simulink model "TEP_Final_NoScript"  (R2024a)
settings: Solver=FixedStepAuto  StartTime=0.0  StopTime=10  FixedStep=1/3600  RelTol=1e-3
model workspace (MAT data in the model file):
  AD : Simulink.Parameter (value not decoded)
  AG : Simulink.Parameter (value not decoded)
  AH : Simulink.Parameter (value not decoded)
  AV : Simulink.Parameter (value not decoded)
  AVP : Simulink.Parameter (value not decoded)
  BCHL : Simulink.Parameter (value not decoded)
  BCHV : Simulink.Parameter (value not decoded)
  BD : Simulink.Parameter (value not decoded)
  BG : Simulink.Parameter (value not decoded)
  BH : Simulink.Parameter (value not decoded)
  BVP : Simulink.Parameter (value not decoded)
  CD : Simulink.Parameter (value not decoded)
  CG : Simulink.Parameter (value not decoded)
  CH : Simulink.Parameter (value not decoded)
  CVP : Simulink.Parameter (value not decoded)
  XMW : Simulink.Parameter (value not decoded)
  XNS : Simulink.Parameter (value not decoded)
  XNSE : Simulink.Parameter (value not decoded)
symbols that are objects in the model workspace (value not decoded): AD, AG, AH, AV, AVP, BD, BG, BH, BVP, CD, CG, CH, CVP, XMW, XNS, XNSE
undefined symbols (not defined in the file or in its folder): magnitude, msgbox, SETPT, XMEAS, XMV
libraries: mylib x360, dspindex x28
(part 5 of 14)

== system TEP_Final_NoScript/Mixing Zone/Holdup of Components in Mixing Zone/Subsystem ==
  Properties of Stream 1 : Inport
  Bus Creator : BusCreator  Inputs=8
  Bus Selector : BusSelector  OutputSignals=FCM(I;1)
  Multiport Selector : dspindex/Multiport Selector  rowsOrCols=Rows  idxCellArray={ 1,2,3,4,5,6,7,8}  idxErrMode=Clip Index
  FCM(I;1) : Outport  VectorParamsAs1DForOutWhenUnconnected=off
  wires:
  Multiport Selector/1 -> Bus Creator/1  "FCM(1;1)"
  Multiport Selector/2 -> Bus Creator/2  "FCM(2;1)"
  Multiport Selector/8 -> Bus Creator/8  "FCM(8;1)"
  Multiport Selector/6 -> Bus Creator/6  "FCM(6;1)"
  Multiport Selector/7 -> Bus Creator/7  "FCM(7;1)"
  Multiport Selector/4 -> Bus Creator/4  "FCM(4;1)"
  Multiport Selector/5 -> Bus Creator/5  "FCM(5;1)"
  Multiport Selector/3 -> Bus Creator/3  "FCM(3;1)"
  Bus Selector/1 -> Multiport Selector/1  "<FCM(I;1)>"
  Properties of Stream 1/1 -> Bus Selector/1
  Bus Creator/1 -> FCM(I;1)/1

== system TEP_Final_NoScript/Mixing Zone/Holdup of Components in Mixing Zone/Subsystem1 ==
  Properties of Stream 2 : Inport
  Bus Creator : BusCreator  Inputs=8
  Bus Selector1 : BusSelector  OutputSignals=FCM(I;2)
  Multiport Selector1 : dspindex/Multiport Selector  rowsOrCols=Rows  idxCellArray={ 1,2,3,4,5,6,7,8}  idxErrMode=Clip Index
  FCM(I;2) : Outport  VectorParamsAs1DForOutWhenUnconnected=off
  wires:
  Multiport Selector1/5 -> Bus Creator/5  "FCM(5;2)"
  Bus Selector1/1 -> Multiport Selector1/1  "<FCM(I;2)>"
  Multiport Selector1/6 -> Bus Creator/6  "FCM(6;2)"
  Multiport Selector1/1 -> Bus Creator/1  "FCM(1;2)"
  Multiport Selector1/2 -> Bus Creator/2  "FCM(2;2)"
  Multiport Selector1/7 -> Bus Creator/7  "FCM(7;2)"
  Multiport Selector1/4 -> Bus Creator/4  "FCM(4;2)"
  Multiport Selector1/8 -> Bus Creator/8  "FCM(8;2)"
  Multiport Selector1/3 -> Bus Creator/3  "FCM(3;2)"
  Properties of Stream 2/1 -> Bus Selector1/1
  Bus Creator/1 -> FCM(I;2)/1

== system TEP_Final_NoScript/Mixing Zone/Holdup of Components in Mixing Zone/Subsystem2 ==
  Bus Creator : BusCreator  Inputs=8
  Bus Selector5 : BusSelector  OutputSignals=signal1.FCM(I;6) = FCM(I;7)
  Multiport Selector4 : dspindex/Multiport Selector  rowsOrCols=Rows  idxCellArray={ 1,2,3,4,5,6,7,8}  idxErrMode=Clip Index
  FCM(I;6) : Outport  VectorParamsAs1DForOutWhenUnconnected=off
  wires:
  Multiport Selector4/6 -> Bus Creator/6  "FCM(6;7)"
  Multiport Selector4/7 -> Bus Creator/7  "FCM(7;7)"
  Multiport Selector4/5 -> Bus Creator/5  "FCM(5;7)"
  Multiport Selector4/4 -> Bus Creator/4  "FCM(4;7)"
  Multiport Selector4/8 -> Bus Creator/8  "FCM(8;7)"
  Multiport Selector4/3 -> Bus Creator/3  "FCM(3;7)"
  Multiport Selector4/2 -> Bus Creator/2  "FCM(2;7)"
  [PropertiesStream6] -> Bus Selector5/1
  Multiport Selector4/1 -> Bus Creator/1  "FCM(1;7)"
  Bus Selector5/1 -> Multiport Selector4/1  "<FCM(I;6) = FCM(I;7)>"
  Bus Creator/1 -> FCM(I;6)/1

== system TEP_Final_NoScript/Mixing Zone/Holdup of Components in Mixing Zone/Subsystem3 ==
  Properties of Stream 3 : Inport
  Bus Creator : BusCreator  Inputs=8
  Bus Selector2 : BusSelector  OutputSignals=FCM(I;3)
  Multiport Selector2 : dspindex/Multiport Selector  rowsOrCols=Rows  idxCellArray={ 1,2,3,4,5,6,7,8}  idxErrMode=Clip Index
  FCM(I;3) : Outport  VectorParamsAs1DForOutWhenUnconnected=off
  wires:
  Multiport Selector2/2 -> Bus Creator/2  "FCM(2;3)"
  Multiport Selector2/4 -> Bus Creator/4  "FCM(4;3)"
  Multiport Selector2/8 -> Bus Creator/8  "FCM(8;3)"
  Bus Selector2/1 -> Multiport Selector2/1  "<FCM(I;3)>"
  Multiport Selector2/7 -> Bus Creator/7  "FCM(7;3)"
  Multiport Selector2/6 -> Bus Creator/6  "FCM(6;3)"
  Multiport Selector2/1 -> Bus Creator/1  "FCM(1;3)"
  Multiport Selector2/3 -> Bus Creator/3  "FCM(3;3)"
  Multiport Selector2/5 -> Bus Creator/5  "FCM(5;3)"
  Properties of Stream 3/1 -> Bus Selector2/1
  Bus Creator/1 -> FCM(I;3)/1

== system TEP_Final_NoScript/Mixing Zone/Holdup of Components in Mixing Zone/Subsystem4 ==
  Properties of Stream 5 : Inport
  Bus Creator : BusCreator  Inputs=8
  Bus Selector3 : BusSelector  OutputSignals=FCM(I;5)
  Multiport Selector3 : dspindex/Multiport Selector  rowsOrCols=Rows  idxCellArray={ 1,2,3,4,5,6,7,8}  idxErrMode=Clip Index
  FCM(I;5) : Outport  VectorParamsAs1DForOutWhenUnconnected=off
  wires:
  Multiport Selector3/6 -> Bus Creator/6  "FCM(6;5)"
  Multiport Selector3/8 -> Bus Creator/8  "FCM(8;5)"
  Multiport Selector3/5 -> Bus Creator/5  "FCM(5;5)"
  Multiport Selector3/2 -> Bus Creator/2  "FCM(2;5)"
  Bus Selector3/1 -> Multiport Selector3/1  "<FCM(I;5)>"
  Multiport Selector3/7 -> Bus Creator/7  "FCM(7;5)"
  Multiport Selector3/4 -> Bus Creator/4  "FCM(4;5)"
  Multiport Selector3/1 -> Bus Creator/1  "FCM(1;5)"
  Multiport Selector3/3 -> Bus Creator/3  "FCM(3;5)"
  Properties of Stream 5/1 -> Bus Selector3/1
  Bus Creator/1 -> FCM(I;5)/1

== system TEP_Final_NoScript/Mixing Zone/Holdup of Components in Mixing Zone/Subsystem5 ==
  Properties of Stream 9 : Inport
  Bus Creator : BusCreator  Inputs=8
  Bus Selector4 : BusSelector  OutputSignals=FCM(I;9)
  Multiport Selector5 : dspindex/Multiport Selector  rowsOrCols=Rows  idxCellArray={ 1,2,3,4,5,6,7,8}  idxErrMode=Clip Index
  FCM(I;9) : Outport  VectorParamsAs1DForOutWhenUnconnected=off
  wires:
  Multiport Selector5/7 -> Bus Creator/7  "FCM(7;9)"
  Multiport Selector5/6 -> Bus Creator/6  "FCM(6;9)"
  Multiport Selector5/8 -> Bus Creator/8  "FCM(8;9)"
  Bus Selector4/1 -> Multiport Selector5/1  "<FCM(I;9)>"
  Multiport Selector5/1 -> Bus Creator/1  "FCM(1;9)"
  Multiport Selector5/2 -> Bus Creator/2  "FCM(2;9)"
  Multiport Selector5/5 -> Bus Creator/5  "FCM(5;9)"
  Multiport Selector5/4 -> Bus Creator/4  "FCM(4;9)"
  Multiport Selector5/3 -> Bus Creator/3  "FCM(3;9)"
  Properties of Stream 9/1 -> Bus Selector4/1
  Bus Creator/1 -> FCM(I;9)/1

== system TEP_Final_NoScript/Mixing Zone/Holdup of Components in Mixing Zone/Vapour Holdup Fraction in the Mxing Zone ==
  UTVV : Inport
  UCVV : Inport  Port=2
  Bus Selector : BusSelector  OutputSignals=UCVV(1),UCVV(2),UCVV(3),UCVV(4),UCVV(5),UCVV(6),UCVV(7),UCVV(8)
  Mux : Mux  Inputs=8
  XVV(1) : Product  Inputs=*/
  XVV(2) : Product  Inputs=*/
  XVV(3) : Product  Inputs=*/
  XVV(4) : Product  Inputs=*/
  XVV(5) : Product  Inputs=*/
  XVV(6) : Product  Inputs=*/
  XVV(7) : Product  Inputs=*/
  XVV(8) : Product  Inputs=*/
  XVV : Outport  VectorParamsAs1DForOutWhenUnconnected=off
  wires:
  XVV(4)/1 -> Mux/4  "XVV(4)"
  UTVV/1 -> XVV(8)/2, XVV(7)/2, XVV(6)/2, XVV(5)/2, XVV(4)/2, XVV(3)/2, XVV(2)/2, XVV(1)/2
  XVV(8)/1 -> Mux/8  "XVV(8)"
  Bus Selector/3 -> XVV(3)/1  "<UCVV(3)>"
  XVV(5)/1 -> Mux/5  "XVV(5)"
  XVV(2)/1 -> Mux/2  "XVV(2)"
  XVV(7)/1 -> Mux/7  "XVV(7)"
  Bus Selector/8 -> XVV(8)/1  "<UCVV(8)>"
  XVV(6)/1 -> Mux/6  "XVV(6)"
  XVV(3)/1 -> Mux/3  "XVV(3)"
  Mux/1 -> XVV/1
  XVV(1)/1 -> Mux/1  "XVV(1)"
  Bus Selector/7 -> XVV(7)/1  "<UCVV(7)>"
  Bus Selector/5 -> XVV(5)/1  "<UCVV(5)>"
  Bus Selector/4 -> XVV(4)/1  "<UCVV(4)>"
  Bus Selector/2 -> XVV(2)/1  "<UCVV(2)>"
  Bus Selector/6 -> XVV(6)/1  "<UCVV(6)>"
  UCVV/1 -> Bus Selector/1
  Bus Selector/1 -> XVV(1)/1  "<UCVV(1)>"

== system TEP_Final_NoScript/Mixing Zone/Holdup of Components in Mixing Zone/YP(28) ==
  FCM(1,1) : Inport
  FCM(1,2) : Inport  Port=2
  FCM(1,3) : Inport  Port=3
  FCM(1,5) : Inport  Port=4
  FCM(1,9) : Inport  Port=5
  FCM(1,6) : Inport  Port=6
  " " : Sum  Inputs=+++++-
  Bus Selector : BusSelector  OutputSignals=FCM(1;1)
  Bus Selector1 : BusSelector  OutputSignals=FCM(1;2)
  Bus Selector2 : BusSelector  OutputSignals=FCM(1;3)
  Bus Selector3 : BusSelector  OutputSignals=FCM(1;5)
  Bus Selector4 : BusSelector  OutputSignals=FCM(1;9)
  Bus Selector5 : BusSelector  OutputSignals=FCM(1;7)
  Integration : mylib/Integration  SystemSampleTime=-1  VariantActivationTime=update diagram  AllowFlexibleInterface=on  Latency=0  AutoFrameSizeCalculation=off
      settings: SourceProductName=TEP Library
  "YY(28) " : Constant  Value=107.7562698
  YY(28) : Outport  VectorParamsAs1DForOutWhenUnconnected=off
  wires:
  "YY(28) "/1 -> Integration/2
  FCM(1,3)/1 -> Bus Selector2/1
  FCM(1,2)/1 -> Bus Selector1/1
  " "/1 -> Integration/1
  Integration/1 -> YY(28)/1
  FCM(1,5)/1 -> Bus Selector3/1
  FCM(1,9)/1 -> Bus Selector4/1
  FCM(1,6)/1 -> Bus Selector5/1
  FCM(1,1)/1 -> Bus Selector/1
  Bus Selector/1 -> " "/1  "<FCM(1;1)>"
  Bus Selector1/1 -> " "/2  "<FCM(1;2)>"
  Bus Selector2/1 -> " "/3  "<FCM(1;3)>"
  Bus Selector3/1 -> " "/4  "<FCM(1;5)>"
  Bus Selector4/1 -> " "/5  "<FCM(1;9)>"
  Bus Selector5/1 -> " "/6  "<FCM(1;7)>"

== system TEP_Final_NoScript/Mixing Zone/Holdup of Components in Mixing Zone/YP(29) ==
  FCM(2,1) : Inport
  FCM(2,2) : Inport  Port=2
  FCM(2,3) : Inport  Port=3
  FCM(2,5) : Inport  Port=4
  FCM(2,9) : Inport  Port=5
  FCM(2,6) : Inport  Port=6
  " " : Sum  Inputs=+++++-
  Bus Selector : BusSelector  OutputSignals=FCM(2;1)
  Bus Selector1 : BusSelector  OutputSignals=FCM(2;2)
  Bus Selector2 : BusSelector  OutputSignals=FCM(2;3)
  Bus Selector3 : BusSelector  OutputSignals=FCM(2;5)
  Bus Selector4 : BusSelector  OutputSignals=FCM(2;9)
  Bus Selector5 : BusSelector  OutputSignals=FCM(2;7)
  Integration : mylib/Integration  SystemSampleTime=-1  VariantActivationTime=update diagram  AllowFlexibleInterface=on  Latency=0  AutoFrameSizeCalculation=off
      settings: SourceProductName=TEP Library
  YY(29)1 : Constant  Value=29.77250546
  YY(29) : Outport  VectorParamsAs1DForOutWhenUnconnected=off
  wires:
  YY(29)1/1 -> Integration/2
  FCM(2,3)/1 -> Bus Selector2/1
  FCM(2,2)/1 -> Bus Selector1/1
  FCM(2,1)/1 -> Bus Selector/1
  " "/1 -> Integration/1
  Integration/1 -> YY(29)/1
  FCM(2,5)/1 -> Bus Selector3/1
  FCM(2,9)/1 -> Bus Selector4/1
  FCM(2,6)/1 -> Bus Selector5/1
  Bus Selector/1 -> " "/1  "<FCM(2;1)>"
  Bus Selector1/1 -> " "/2  "<FCM(2;2)>"
  Bus Selector2/1 -> " "/3  "<FCM(2;3)>"
  Bus Selector3/1 -> " "/4  "<FCM(2;5)>"
  Bus Selector4/1 -> " "/5  "<FCM(2;9)>"
  Bus Selector5/1 -> " "/6  "<FCM(2;7)>"

== system TEP_Final_NoScript/Mixing Zone/Holdup of Components in Mixing Zone/YP(30) ==
  FCM(3,1) : Inport
  FCM(3,2) : Inport  Port=2
  FCM(3,3) : Inport  Port=3
  FCM(3,5) : Inport  Port=4
  FCM(3,9) : Inport  Port=5
  FCM(3,6) : Inport  Port=6
  " " : Sum  Inputs=+++++-
  Bus Selector : BusSelector  OutputSignals=FCM(3;1)
  Bus Selector1 : BusSelector  OutputSignals=FCM(3;2)
  Bus Selector2 : BusSelector  OutputSignals=FCM(3;3)
  Bus Selector3 : BusSelector  OutputSignals=FCM(3;5)
  Bus Selector4 : BusSelector  OutputSignals=FCM(3;9)
  Bus Selector5 : BusSelector  OutputSignals=FCM(3;7)
  Integration : mylib/Integration  SystemSampleTime=-1  VariantActivationTime=update diagram  AllowFlexibleInterface=on  Latency=0  AutoFrameSizeCalculation=off
      settings: SourceProductName=TEP Library
  YY(30)1 : Constant  Value=88.32481135
  YY(30) : Outport  VectorParamsAs1DForOutWhenUnconnected=off
  wires:
  YY(30)1/1 -> Integration/2
  FCM(3,3)/1 -> Bus Selector2/1
  FCM(3,2)/1 -> Bus Selector1/1
  FCM(3,1)/1 -> Bus Selector/1
  " "/1 -> Integration/1
  Integration/1 -> YY(30)/1
  FCM(3,5)/1 -> Bus Selector3/1
  FCM(3,9)/1 -> Bus Selector4/1
  FCM(3,6)/1 -> Bus Selector5/1
  Bus Selector/1 -> " "/1  "<FCM(3;1)>"
  Bus Selector1/1 -> " "/2  "<FCM(3;2)>"
  Bus Selector2/1 -> " "/3  "<FCM(3;3)>"
  Bus Selector3/1 -> " "/4  "<FCM(3;5)>"
  Bus Selector4/1 -> " "/5  "<FCM(3;9)>"
  Bus Selector5/1 -> " "/6  "<FCM(3;7)>"

== system TEP_Final_NoScript/Mixing Zone/Holdup of Components in Mixing Zone/YP(31) ==
  FCM(4,1) : Inport
  FCM(4,2) : Inport  Port=2
  FCM(4,3) : Inport  Port=3
  FCM(4,5) : Inport  Port=4
  FCM(4,9) : Inport  Port=5
  FCM(4,6) : Inport  Port=6
  " " : Sum  Inputs=+++++-
  Bus Selector : BusSelector  OutputSignals=FCM(4;1)
  Bus Selector1 : BusSelector  OutputSignals=FCM(4;2)
  Bus Selector2 : BusSelector  OutputSignals=FCM(4;3)
  Bus Selector3 : BusSelector  OutputSignals=FCM(4;5)
  Bus Selector4 : BusSelector  OutputSignals=FCM(4;9)
  Bus Selector5 : BusSelector  OutputSignals=FCM(4;7)
  Integration : mylib/Integration  SystemSampleTime=-1  VariantActivationTime=update diagram  AllowFlexibleInterface=on  Latency=0  AutoFrameSizeCalculation=off
      settings: SourceProductName=TEP Library
  YY(31)1 : Constant  Value=23.03929507
  YY(31) : Outport  VectorParamsAs1DForOutWhenUnconnected=off
  wires:
  YY(31)1/1 -> Integration/2
  FCM(4,3)/1 -> Bus Selector2/1
  FCM(4,2)/1 -> Bus Selector1/1
  FCM(4,1)/1 -> Bus Selector/1
  " "/1 -> Integration/1
  Integration/1 -> YY(31)/1
  FCM(4,5)/1 -> Bus Selector3/1
  FCM(4,9)/1 -> Bus Selector4/1
  FCM(4,6)/1 -> Bus Selector5/1
  Bus Selector/1 -> " "/1  "<FCM(4;1)>"
  Bus Selector1/1 -> " "/2  "<FCM(4;2)>"
  Bus Selector2/1 -> " "/3  "<FCM(4;3)>"
  Bus Selector3/1 -> " "/4  "<FCM(4;5)>"
  Bus Selector4/1 -> " "/5  "<FCM(4;9)>"
  Bus Selector5/1 -> " "/6  "<FCM(4;7)>"

== system TEP_Final_NoScript/Mixing Zone/Holdup of Components in Mixing Zone/YP(32) ==
  FCM(5,1) : Inport
  FCM(5,2) : Inport  Port=2
  FCM(5,3) : Inport  Port=3
  FCM(5,5) : Inport  Port=4
  FCM(5,9) : Inport  Port=5
  FCM(5,6) : Inport  Port=6
  " " : Sum  Inputs=+++++-
  Bus Selector : BusSelector  OutputSignals=FCM(5;1)
  Bus Selector1 : BusSelector  OutputSignals=FCM(5;2)
  Bus Selector2 : BusSelector  OutputSignals=FCM(5;3)
  Bus Selector3 : BusSelector  OutputSignals=FCM(5;5)
  Bus Selector4 : BusSelector  OutputSignals=FCM(5;9)
  Bus Selector5 : BusSelector  OutputSignals=FCM(5;7)
  Integration : mylib/Integration  SystemSampleTime=-1  VariantActivationTime=update diagram  AllowFlexibleInterface=on  Latency=0  AutoFrameSizeCalculation=off
      settings: SourceProductName=TEP Library
  YY(32)1 : Constant  Value=62.85848794
  YY(32) : Outport  VectorParamsAs1DForOutWhenUnconnected=off
  wires:
  YY(32)1/1 -> Integration/2
  FCM(5,3)/1 -> Bus Selector2/1
  FCM(5,2)/1 -> Bus Selector1/1
  FCM(5,1)/1 -> Bus Selector/1
  " "/1 -> Integration/1
  Integration/1 -> YY(32)/1
  FCM(5,5)/1 -> Bus Selector3/1
  FCM(5,9)/1 -> Bus Selector4/1
  FCM(5,6)/1 -> Bus Selector5/1
  Bus Selector/1 -> " "/1  "<FCM(5;1)>"
  Bus Selector1/1 -> " "/2  "<FCM(5;2)>"
  Bus Selector2/1 -> " "/3  "<FCM(5;3)>"
  Bus Selector3/1 -> " "/4  "<FCM(5;5)>"
  Bus Selector4/1 -> " "/5  "<FCM(5;9)>"
  Bus Selector5/1 -> " "/6  "<FCM(5;7)>"

== system TEP_Final_NoScript/Mixing Zone/Holdup of Components in Mixing Zone/YP(33) ==
  FCM(6,1) : Inport
  FCM(6,2) : Inport  Port=2
  FCM(6,3) : Inport  Port=3
  FCM(6,5) : Inport  Port=4
  FCM(6,9) : Inport  Port=5
  FCM(6,6) : Inport  Port=6
  " " : Sum  Inputs=+++++-
  Bus Selector : BusSelector  OutputSignals=FCM(6;1)
  Bus Selector1 : BusSelector  OutputSignals=FCM(6;2)
  Bus Selector2 : BusSelector  OutputSignals=FCM(6;3)
  Bus Selector3 : BusSelector  OutputSignals=FCM(6;5)
  Bus Selector4 : BusSelector  OutputSignals=FCM(6;9)
  Bus Selector5 : BusSelector  OutputSignals=FCM(6;7)
  Integration : mylib/Integration  SystemSampleTime=-1  VariantActivationTime=update diagram  AllowFlexibleInterface=on  Latency=0  AutoFrameSizeCalculation=off
      settings: SourceProductName=TEP Library
  YY(33)1 : Constant  Value=5.546318688
  YY(33) : Outport  VectorParamsAs1DForOutWhenUnconnected=off
  wires:
  YY(33)1/1 -> Integration/2
  FCM(6,3)/1 -> Bus Selector2/1
  FCM(6,2)/1 -> Bus Selector1/1
  FCM(6,1)/1 -> Bus Selector/1
  " "/1 -> Integration/1
  Integration/1 -> YY(33)/1
  FCM(6,5)/1 -> Bus Selector3/1
  FCM(6,9)/1 -> Bus Selector4/1
  FCM(6,6)/1 -> Bus Selector5/1
  Bus Selector/1 -> " "/1  "<FCM(6;1)>"
  Bus Selector1/1 -> " "/2  "<FCM(6;2)>"
  Bus Selector2/1 -> " "/3  "<FCM(6;3)>"
  Bus Selector3/1 -> " "/4  "<FCM(6;5)>"
  Bus Selector4/1 -> " "/5  "<FCM(6;9)>"
  Bus Selector5/1 -> " "/6  "<FCM(6;7)>"

== system TEP_Final_NoScript/Mixing Zone/Holdup of Components in Mixing Zone/YP(34) ==
  FCM(7,1) : Inport
  FCM(7,2) : Inport  Port=2
  FCM(7,3) : Inport  Port=3
  FCM(7,5) : Inport  Port=4
  FCM(7,9) : Inport  Port=5
  FCM(7,6) : Inport  Port=6
  " " : Sum  Inputs=+++++-
  Bus Selector : BusSelector  OutputSignals=FCM(7;1)
  Bus Selector1 : BusSelector  OutputSignals=FCM(7;2)
  Bus Selector2 : BusSelector  OutputSignals=FCM(7;3)
  Bus Selector3 : BusSelector  OutputSignals=FCM(7;5)
  Bus Selector4 : BusSelector  OutputSignals=FCM(7;9)
  Bus Selector5 : BusSelector  OutputSignals=FCM(7;7)
  Integration : mylib/Integration  SystemSampleTime=-1  VariantActivationTime=update diagram  AllowFlexibleInterface=on  Latency=0  AutoFrameSizeCalculation=off
      settings: SourceProductName=TEP Library
  YY(34)1 : Constant  Value=11.92244772
  YY(34) : Outport  VectorParamsAs1DForOutWhenUnconnected=off
  wires:
  YY(34)1/1 -> Integration/2
  FCM(7,3)/1 -> Bus Selector2/1
  FCM(7,2)/1 -> Bus Selector1/1
  FCM(7,1)/1 -> Bus Selector/1
  " "/1 -> Integration/1
  Integration/1 -> YY(34)/1
  FCM(7,5)/1 -> Bus Selector3/1
  FCM(7,9)/1 -> Bus Selector4/1
  FCM(7,6)/1 -> Bus Selector5/1
  Bus Selector/1 -> " "/1  "<FCM(7;1)>"
  Bus Selector1/1 -> " "/2  "<FCM(7;2)>"
  Bus Selector2/1 -> " "/3  "<FCM(7;3)>"
  Bus Selector3/1 -> " "/4  "<FCM(7;5)>"
  Bus Selector4/1 -> " "/5  "<FCM(7;9)>"
  Bus Selector5/1 -> " "/6  "<FCM(7;7)>"

== system TEP_Final_NoScript/Mixing Zone/Holdup of Components in Mixing Zone/YP(35) ==
  FCM(8,1) : Inport
  FCM(8,2) : Inport  Port=2
  FCM(8,3) : Inport  Port=3
  FCM(8,5) : Inport  Port=4
  FCM(8,9) : Inport  Port=5
  FCM(8,6) : Inport  Port=6
  " " : Sum  Inputs=+++++-
  Bus Selector : BusSelector  OutputSignals=FCM(8;1)
  Bus Selector1 : BusSelector  OutputSignals=FCM(8;2)
  Bus Selector2 : BusSelector  OutputSignals=FCM(8;3)
  Bus Selector3 : BusSelector  OutputSignals=FCM(8;5)
  Bus Selector4 : BusSelector  OutputSignals=FCM(8;9)
  Bus Selector5 : BusSelector  OutputSignals=FCM(8;7)
  Integration : mylib/Integration  SystemSampleTime=-1  VariantActivationTime=update diagram  AllowFlexibleInterface=on  Latency=0  AutoFrameSizeCalculation=off
      settings: SourceProductName=TEP Library
  YY(35)1 : Constant  Value=5.555448243
  YY(35) : Outport  VectorParamsAs1DForOutWhenUnconnected=off
  wires:
  YY(35)1/1 -> Integration/2
  FCM(8,3)/1 -> Bus Selector2/1
  FCM(8,2)/1 -> Bus Selector1/1
  FCM(8,1)/1 -> Bus Selector/1
  " "/1 -> Integration/1
  Integration/1 -> YY(35)/1
  FCM(8,5)/1 -> Bus Selector3/1
  FCM(8,9)/1 -> Bus Selector4/1
  FCM(8,6)/1 -> Bus Selector5/1
  Bus Selector/1 -> " "/1  "<FCM(8;1)>"
  Bus Selector1/1 -> " "/2  "<FCM(8;2)>"
  Bus Selector2/1 -> " "/3  "<FCM(8;3)>"
  Bus Selector3/1 -> " "/4  "<FCM(8;5)>"
  Bus Selector4/1 -> " "/5  "<FCM(8;9)>"
  Bus Selector5/1 -> " "/6  "<FCM(8;7)>"

== system TEP_Final_NoScript/Mixing Zone/Stream 6/HST(6) Molar Enthalpy of Stream 6 MBtu//lb-mol ==
  ITY : Inport
  T : Inport  Port=2
  XST(I,6) : Inport  Port=3
  "Enthalpy of Stream " : mylib/Enthalpy of Stream   SystemSampleTime=-1  VariantActivationTime=update diagram  AllowFlexibleInterface=on  Latency=0  AutoFrameSizeCalculation=off
      settings: SourceProductName=TEP Library
  "H " : Outport  VectorParamsAs1DForOutWhenUnconnected=off
  wires:
  ITY/1 -> "Enthalpy of Stream "/1
  T/1 -> "Enthalpy of Stream "/2
  XST(I,6)/1 -> "Enthalpy of Stream "/3
  "Enthalpy of Stream "/1 -> "H "/1

== system TEP_Final_NoScript/Mixing Zone/Stream 6/Subsystem ==
  Abs : Abs  SaturateOnIntegerOverflow=off
  Constant : Constant  Value=0.0
  Constant1 : Constant  Value=1937.6
  DLP : Sum  Inputs=+-
  DLP Pressure drop between reactor and mixing zone : Merge
  FLMS : Product
  If : If  IfExpression=u1 < 0
  If Action Subsystem : Subsystem  TreatAsAtomicUnit=on
  If Action Subsystem1 : Subsystem  TreatAsAtomicUnit=on
  Sqrt : Sqrt
  "FLMS " : Outport  VectorParamsAs1DForOutWhenUnconnected=off
  wires:
  [PTR] -> DLP/2
  Abs/1 -> Sqrt/1
  Constant1/1 -> FLMS/1
  If Action Subsystem/1(Out1) -> DLP Pressure drop between reactor and mixing zone/1
  If Action Subsystem1/1(Out1) -> DLP Pressure drop between reactor and mixing zone/2
  [PTV] -> DLP/1
  Constant/1 -> If Action Subsystem/1(In1)
  Sqrt/1 -> FLMS/2
  DLP/1 -> If Action Subsystem1/1(In1), If/1
  If/1 -> If Action Subsystem/Action
  DLP Pressure drop between reactor and mixing zone/1 -> Abs/1
  If/2 -> If Action Subsystem1/Action
  FLMS/1 -> "FLMS "/1

== system TEP_Final_NoScript/Mixing Zone/Stream 6/XMWS(6) Molecular weight of Stream 6 lb//lb-mol ==
  XST(I,6) : Inport
  Product : Product
  Sum of Elements : Sum  Inputs=+
  "XMW(I) Molecular weight of components lb/lb-mol " : Constant  Value=XMW
  XMWS(6) : Outport  VectorParamsAs1DForOutWhenUnconnected=off
  wires:
  Sum of Elements/1 -> XMWS(6)/1
  Product/1 -> Sum of Elements/1
  XST(I,6)/1 -> Product/1
  "XMW(I) Molecular weight of components lb/lb-mol "/1 -> Product/2

== system TEP_Final_NoScript/Process Measurements/Feed Streams/ A Feed ==
  " " : Constant  Value=35.3145
  "  " : Constant  Value=0.359
  Add : Sum
  Bus Selector : BusSelector  OutputSignals=FTM(3)
  Bus Selector1 : BusSelector  OutputSignals=XMNS(1)
  Display : Display
  Display1 : Display
  Display2 : Display
  Product1 : Product  Inputs=**/
  "XMEAS(1) " : Outport  PortDimensions=1  VectorParamsAs1DForOutWhenUnconnected=off
  wires:
  " "/1 -> Product1/3
  "  "/1 -> Product1/2
  [PropertiesStream3] -> Bus Selector/1
  Bus Selector/1 -> Product1/1  "<FTM(3)>"
  Product1/1 -> Display/1, Add/1
  Add/1 -> Display1/1, "XMEAS(1) "/1  "XMEAS(1)"
  [XMNS] -> Bus Selector1/1
  Bus Selector1/1 -> Add/2, Display2/1  "<XMNS(1)>"

== system TEP_Final_NoScript/Process Measurements/Feed Streams/A and C Feed ==
  " " : Constant  Value=35.3145
  "  " : Constant  Value=0.359
  Add : Sum
  Bus Selector : BusSelector  OutputSignals=FTM(4)
  Bus Selector1 : BusSelector  OutputSignals=XMNS(4)
  Product1 : Product  Inputs=**/
  "XMEAS(4) " : Outport  PortDimensions=1  VectorParamsAs1DForOutWhenUnconnected=off
  wires:
  " "/1 -> Product1/3
  "  "/1 -> Product1/2
  [PropertiesStream4] -> Bus Selector/1
  Bus Selector/1 -> Product1/1  "<FTM(4)>"
  Bus Selector1/1 -> Add/2  "<XMNS(4)>"
  Product1/1 -> Add/1
  Add/1 -> "XMEAS(4) "/1  "XMEAS(4)"
  [XMNS] -> Bus Selector1/1

== system TEP_Final_NoScript/Process Measurements/Feed Streams/D Feed ==
  Add : Sum
  Bus Selector : BusSelector  OutputSignals=XST(I;1),FTM(1)
  Bus Selector1 : BusSelector  OutputSignals=XMNS(2)
  Convert from lb/h to kg/h : Constant  Value=0.454
  Product : Product  Inputs=3
  XMWS(1) Molecular weight of Stream 1 lb/lb-mol : Subsystem
  "XMEAS(2) " : Outport  VectorParamsAs1DForOutWhenUnconnected=off
  wires:
  Convert from lb/h to kg/h/1 -> Product/3
  XMWS(1) Molecular weight of Stream 1 lb/lb-mol/1(XMWS(1)) -> Product/1
  [PropertiesStream1] -> Bus Selector/1
  Bus Selector/2 -> Product/2  "<FTM(1)>"
  Bus Selector/1 -> XMWS(1) Molecular weight of Stream 1 lb/lb-mol/1(XST(I,1))  "<XST(I;1)>"
  Bus Selector1/1 -> Add/2  "<XMNS(2)>"
  Product/1 -> Add/1
  Add/1 -> "XMEAS(2) "/1  "XMEAS(2)"
  [XMNS] -> Bus Selector1/1

== system TEP_Final_NoScript/Process Measurements/Feed Streams/E Feed ==
  Add : Sum
  Bus Selector : BusSelector  OutputSignals=XST(I;2),FTM(2)
  Bus Selector1 : BusSelector  OutputSignals=XMNS(3)
  Convert from lb/h to kg/h : Constant  Value=0.454
  Product : Product  Inputs=3
  XMWS(2) Molecular weight of Stream 2 lb/lb-mol : Subsystem
  "XMEAS(3) " : Outport  VectorParamsAs1DForOutWhenUnconnected=off
  wires:
  Convert from lb/h to kg/h/1 -> Product/3
  Bus Selector/1 -> XMWS(2) Molecular weight of Stream 2 lb/lb-mol/1(XST(I,2))  "<XST(I;2)>"
  XMWS(2) Molecular weight of Stream 2 lb/lb-mol/1(XMWS(2)) -> Product/1
  Bus Selector/2 -> Product/2  "<FTM(2)>"
  [PropertiesStream2] -> Bus Selector/1
  Bus Selector1/1 -> Add/2  "<XMNS(3)>"
  Product/1 -> Add/1
  Add/1 -> "XMEAS(3) "/1  "XMEAS(3)"
  [XMNS] -> Bus Selector1/1

== system TEP_Final_NoScript/Process Measurements/Feed Streams/Recycle Flow ==
  " " : Constant  Value=35.3145
  "  " : Constant  Value=0.359
  Add : Sum
  Bus Selector : BusSelector  OutputSignals=signal2.FTM(9)
  Bus Selector1 : BusSelector  OutputSignals=XMNS(5)
  Product1 : Product  Inputs=**/
  "XMEAS(5) " : Outport  VectorParamsAs1DForOutWhenUnconnected=off
  wires:
  " "/1 -> Product1/3
  Bus Selector/1 -> Product1/1  "<FTM(9)>"
  "  "/1 -> Product1/2
  [PropertiesStream9] -> Bus Selector/1
  Bus Selector1/1 -> Add/2  "<XMNS(5)>"
  Product1/1 -> Add/1
  Add/1 -> "XMEAS(5) "/1  "XMEAS(5)"
  [XMNS] -> Bus Selector1/1

== system TEP_Final_NoScript/Process Measurements/Product analysis/Subsystem ==
  <XST(I;13)> : Inport
  Bus Selector : BusSelector  OutputSignals=XMNS(37),XMNS(38),XMNS(39),XMNS(40),XMNS(41)
  Process Noise I=37-{1..4,41} (5 alike) : mylib/Process Noise I=37-41  SystemSampleTime=-1  VariantActivationTime=update diagram  AllowFlexibleInterface=on  Latency=0  AutoFrameSizeCalculation=off
      settings: SourceProductName=TEP Library
  Subsystem : Subsystem
  XMEAS(37) : Outport  VectorParamsAs1DForOutWhenUnconnected=off
  XMEAS(38) : Outport  Port=2  VectorParamsAs1DForOutWhenUnconnected=off
  XMEAS(39) : Outport  Port=3  VectorParamsAs1DForOutWhenUnconnected=off
  XMEAS(40) : Outport  Port=4  VectorParamsAs1DForOutWhenUnconnected=off
  XMEAS(41) : Outport  Port=5  VectorParamsAs1DForOutWhenUnconnected=off
  wires:
  Process Noise I=37-41/1 -> XMEAS(37)/1
  Bus Selector/1 -> Process Noise I=37-41/2  "<XMNS(37)>"
  Process Noise I=37-1/1 -> XMEAS(38)/1
  Bus Selector/2 -> Process Noise I=37-1/2  "<XMNS(38)>"
  Process Noise I=37-2/1 -> XMEAS(39)/1
  Bus Selector/3 -> Process Noise I=37-2/2  "<XMNS(39)>"
  Process Noise I=37-3/1 -> XMEAS(40)/1
  Bus Selector/4 -> Process Noise I=37-3/2  "<XMNS(40)>"
  Process Noise I=37-4/1 -> XMEAS(41)/1
  Bus Selector/5 -> Process Noise I=37-4/2  "<XMNS(41)>"
  <XST(I;13)>/1 -> Subsystem/1(XST)
  Subsystem/1("XCMP(37) ") -> Process Noise I=37-41/1
  Subsystem/2("XCMP(38) ") -> Process Noise I=37-1/1
  Subsystem/3("XCMP(39) ") -> Process Noise I=37-2/1
  Subsystem/4("XCMP(40) ") -> Process Noise I=37-3/1
  Subsystem/5("XCMP(41) ") -> Process Noise I=37-4/1
  [XMNS3] -> Bus Selector/1

== system TEP_Final_NoScript/Process Measurements/Purge gas analysis/Subsystem ==
  <XST(I;10)> : Inport
  Bus Selector : BusSelector  OutputSignals=signal2.XMNS(29),signal2.XMNS(30),signal2.XMNS(31),signal2.XMNS(32),signal3.XMNS(33),signal3.XMNS(34),signal3.XMNS(35),signal3.XMNS(36)
  Process Noise I=23-{1..7,36} (8 alike) : mylib/Process Noise I=23-36  SystemSampleTime=-1  VariantActivationTime=update diagram  AllowFlexibleInterface=on  Latency=0  AutoFrameSizeCalculation=off
      settings: SourceProductName=TEP Library
  Subsystem : Subsystem
  XMEAS(29) : Outport  VectorParamsAs1DForOutWhenUnconnected=off
  XMEAS(30) : Outport  Port=2  VectorParamsAs1DForOutWhenUnconnected=off
  XMEAS(31) : Outport  Port=3  VectorParamsAs1DForOutWhenUnconnected=off
  XMEAS(32) : Outport  Port=4  VectorParamsAs1DForOutWhenUnconnected=off
  XMEAS(33) : Outport  Port=5  VectorParamsAs1DForOutWhenUnconnected=off
  XMEAS(34) : Outport  Port=6  VectorParamsAs1DForOutWhenUnconnected=off
  XMEAS(35) : Outport  Port=7  VectorParamsAs1DForOutWhenUnconnected=off
  XMEAS(36) : Outport  Port=8  VectorParamsAs1DForOutWhenUnconnected=off
  wires:
  Process Noise I=23-36/1 -> XMEAS(29)/1
  Process Noise I=23-1/1 -> XMEAS(30)/1
  Bus Selector/2 -> Process Noise I=23-1/2  "<XMNS(30)>"
  Process Noise I=23-2/1 -> XMEAS(31)/1
  Process Noise I=23-3/1 -> XMEAS(32)/1
  Process Noise I=23-4/1 -> XMEAS(33)/1
  Process Noise I=23-5/1 -> XMEAS(34)/1
  Process Noise I=23-6/1 -> XMEAS(35)/1
  Process Noise I=23-7/1 -> XMEAS(36)/1
  Bus Selector/7 -> Process Noise I=23-6/2  "<XMNS(35)>"
  Bus Selector/8 -> Process Noise I=23-7/2  "<XMNS(36)>"
  Bus Selector/6 -> Process Noise I=23-5/2  "<XMNS(34)>"
  Bus Selector/5 -> Process Noise I=23-4/2  "<XMNS(33)>"
  Bus Selector/4 -> Process Noise I=23-3/2  "<XMNS(32)>"
  Bus Selector/3 -> Process Noise I=23-2/2  "<XMNS(31)>"
  Bus Selector/1 -> Process Noise I=23-36/2  "<XMNS(29)>"
  <XST(I;10)>/1 -> Subsystem/1(XST)
  Subsystem/1("XCMP(29) ") -> Process Noise I=23-36/1
  Subsystem/2("XCMP(30) ") -> Process Noise I=23-1/1
  Subsystem/3("XCMP(31) ") -> Process Noise I=23-2/1
  Subsystem/4("XCMP(32) ") -> Process Noise I=23-3/1
  Subsystem/5("XCMP(33) ") -> Process Noise I=23-4/1
  Subsystem/6("XCMP(34) ") -> Process Noise I=23-5/1
  Subsystem/7("XCMP(35) ") -> Process Noise I=23-6/1
  Subsystem/8("XCMP(36) ") -> Process Noise I=23-7/1
  [XMNS2] -> Bus Selector/1

== system TEP_Final_NoScript/Process Measurements/Reactor feed analysis/Subsystem ==
  <XST(I;6) = XST(I;7)> : Inport
  Bus Selector : BusSelector  OutputSignals=signal1.XMNS(23),signal1.XMNS(24),signal1.XMNS(25),signal1.XMNS(26),signal1.XMNS(27),signal2.XMNS(28)
  Process Noise I=23-{1..5,36} (6 alike) : mylib/Process Noise I=23-36  SystemSampleTime=-1  VariantActivationTime=update diagram  AllowFlexibleInterface=on  Latency=0  AutoFrameSizeCalculation=off
      settings: SourceProductName=TEP Library
  Subsystem : Subsystem
  XMEAS(23) : Outport  VectorParamsAs1DForOutWhenUnconnected=off
  XMEAS(24) : Outport  Port=2  VectorParamsAs1DForOutWhenUnconnected=off
  XMEAS(25) : Outport  Port=3  VectorParamsAs1DForOutWhenUnconnected=off
  XMEAS(26) : Outport  Port=4  VectorParamsAs1DForOutWhenUnconnected=off
  XMEAS(27) : Outport  Port=5  VectorParamsAs1DForOutWhenUnconnected=off
  XMEAS(28) : Outport  Port=6  VectorParamsAs1DForOutWhenUnconnected=off
  wires:
  Process Noise I=23-36/1 -> XMEAS(23)/1
  Bus Selector/1 -> Process Noise I=23-36/2  "<XMNS(23)>"
  Process Noise I=23-1/1 -> XMEAS(24)/1
  Process Noise I=23-2/1 -> XMEAS(25)/1
  Process Noise I=23-3/1 -> XMEAS(26)/1
  Process Noise I=23-4/1 -> XMEAS(27)/1
  Process Noise I=23-5/1 -> XMEAS(28)/1
  Bus Selector/2 -> Process Noise I=23-1/2  "<XMNS(24)>"
  Bus Selector/3 -> Process Noise I=23-2/2  "<XMNS(25)>"
  Bus Selector/4 -> Process Noise I=23-3/2  "<XMNS(26)>"
  Bus Selector/6 -> Process Noise I=23-5/2  "<XMNS(28)>"
  <XST(I;6) = XST(I;7)>/1 -> Subsystem/1(XST)
  Subsystem/1(XCMP(23)1) -> Process Noise I=23-36/1
  Subsystem/2(XCMP(24)1) -> Process Noise I=23-1/1
  Subsystem/3(XCMP(25)1) -> Process Noise I=23-2/1
  Subsystem/4(XCMP(26)1) -> Process Noise I=23-3/1
  Subsystem/5(XCMP(27)1) -> Process Noise I=23-4/1
  Subsystem/6(XCMP(28)1) -> Process Noise I=23-5/1
  [XMNS2] -> Bus Selector/1
  Bus Selector/5 -> Process Noise I=23-4/2  "<XMNS(27)>"

== system TEP_Final_NoScript/Process Measurements/Subsystem3/Reactor Feed  ==
  " " : Constant  Value=35.3145
  "  " : Constant  Value=0.359
  Add : Sum
  Bus Selector : BusSelector  OutputSignals=signal1.FTM(6) = FTM(7)
  Bus Selector1 : BusSelector  OutputSignals=XMNS(6)
  Product1 : Product  Inputs=**/
  "XMEAS(6) " : Outport  VectorParamsAs1DForOutWhenUnconnected=off
  wires:
  " "/1 -> Product1/3
  "  "/1 -> Product1/2
  [PropertiesStream6] -> Bus Selector/1
  Bus Selector/1 -> Product1/1  "<FTM(6) = FTM(7)>"
  Product1/1 -> Add/1
  Add/1 -> "XMEAS(6) "/1  "XMEAS(6)"
  Bus Selector1/1 -> Add/2  "<XMNS(6)>"
  [XMNS] -> Bus Selector1/1

== system TEP_Final_NoScript/Process Measurements/Subsystem3/Reactor Level ==
  " " : Sum  Inputs=+-
  "    " : Constant  Value=84.6
  "      " : Constant  Value=666.7
  "       " : Constant  Value=100
  Add : Sum
  Bus Selector1 : BusSelector  OutputSignals=XMNS(8)
  XMEAS(8) : Product  Inputs=*/*
  "XMEAS(8) " : Outport  VectorParamsAs1DForOutWhenUnconnected=off
  wires:
  " "/1 -> XMEAS(8)/1
  "       "/1 -> XMEAS(8)/3
  "    "/1 -> " "/2
  [VLR] -> " "/1
  "      "/1 -> XMEAS(8)/2
  XMEAS(8)/1 -> Add/1
  Add/1 -> "XMEAS(8) "/1  "XMEAS(8)"
  Bus Selector1/1 -> Add/2  "<XMNS(8)>"
  [XMNS] -> Bus Selector1/1

== system TEP_Final_NoScript/Process Measurements/Subsystem3/Reactor Pressure ==
  " " : Sum  Inputs=+-
  "    " : Constant  Value=760
  "       " : Constant  Value=101.325
  Add : Sum
  Bus Selector1 : BusSelector  OutputSignals=XMNS(7)
  XMEAS(7) : Product  Inputs=*/*
  "XMEAS(7) " : Outport  VectorParamsAs1DForOutWhenUnconnected=off
  wires:
  " "/1 -> XMEAS(7)/1
  "       "/1 -> XMEAS(7)/3
  "    "/1 -> XMEAS(7)/2, " "/2
  [PTR] -> " "/1
  XMEAS(7)/1 -> Add/1
  Add/1 -> "XMEAS(7) "/1  "XMEAS(7)"
  Bus Selector1/1 -> Add/2  "<XMNS(7)>"
  [XMNS] -> Bus Selector1/1

== system TEP_Final_NoScript/Process Measurements/Subsystem3/Reactor Temperature ==
  Add : Sum
  Bus Selector1 : BusSelector  OutputSignals=XMNS(9)
  "XMEAS(9) " : Outport  VectorParamsAs1DForOutWhenUnconnected=off
  wires:
  [TCR] -> Add/1
  Add/1 -> "XMEAS(9) "/1  "XMEAS(9)"
  Bus Selector1/1 -> Add/2  "<XMNS(9)>"
  [XMNS] -> Bus Selector1/1

== system TEP_Final_NoScript/Process Measurements/Subsystem4/Purge Rate ==
  " " : Constant  Value=35.3145
  "  " : Constant  Value=0.359
  Add : Sum
  Bus Selector : BusSelector  OutputSignals=signal1.FTM(10)
  Bus Selector1 : BusSelector  OutputSignals=XMNS(10)
  Product1 : Product  Inputs=**/
  "XMEAS(10) " : Outport  VectorParamsAs1DForOutWhenUnconnected=off
  wires:
  " "/1 -> Product1/3
  Bus Selector/1 -> Product1/1  "<FTM(10)>"
  "  "/1 -> Product1/2
  [PropertiesStream10] -> Bus Selector/1
  Product1/1 -> Add/1
  Add/1 -> "XMEAS(10) "/1  "XMEAS(10)"
  Bus Selector1/1 -> Add/2  "<XMNS(10)>"
  [XMNS] -> Bus Selector1/1

== system TEP_Final_NoScript/Process Measurements/Subsystem4/Separator Level ==
  " " : Sum  Inputs=+-
  "    " : Constant  Value=27.5
  "      " : Constant  Value=290
  "       " : Constant  Value=100
  Add : Sum
  Bus Selector1 : BusSelector  OutputSignals=XMNS(12)
  XMEAS(12) : Product  Inputs=*/*
  "XMEAS(12) " : Outport  VectorParamsAs1DForOutWhenUnconnected=off
  wires:
  " "/1 -> XMEAS(12)/1
  "       "/1 -> XMEAS(12)/3
  "    "/1 -> " "/2
  [VLS] -> " "/1
  "      "/1 -> XMEAS(12)/2
  XMEAS(12)/1 -> Add/1
  Add/1 -> "XMEAS(12) "/1  "XMEAS(12)"
  [XMNS] -> Bus Selector1/1
  Bus Selector1/1 -> Add/2  "<XMNS(12)>"

== system TEP_Final_NoScript/Process Measurements/Subsystem4/Separator Pressure ==
  "       1" : Constant  Value=101.325
  "    1" : Constant  Value=760
  " 1" : Sum  Inputs=+-
  Add : Sum
  Bus Selector1 : BusSelector  OutputSignals=XMNS(13)
  XMEAS(13) : Product  Inputs=*/*
  "XMEAS(13) " : Outport  VectorParamsAs1DForOutWhenUnconnected=off
  wires:
  "       1"/1 -> XMEAS(13)/3
  "    1"/1 -> XMEAS(13)/2, " 1"/2
  " 1"/1 -> XMEAS(13)/1
  [PTS] -> " 1"/1
  XMEAS(13)/1 -> Add/1
  Add/1 -> "XMEAS(13) "/1  "XMEAS(13)"
  [XMNS] -> Bus Selector1/1
  Bus Selector1/1 -> Add/2  "<XMNS(13)>"

== system TEP_Final_NoScript/Process Measurements/Subsystem4/Separator Temperature ==
  Add : Sum
  Bus Selector1 : BusSelector  OutputSignals=XMNS(11)
  "XMEAS(11) " : Outport  VectorParamsAs1DForOutWhenUnconnected=off
  wires:
  [TCS] -> Add/1
  Add/1 -> "XMEAS(11) "/1  "XMEAS(11)"
  [XMNS] -> Bus Selector1/1
  Bus Selector1/1 -> Add/2  "<XMNS(11)>"

== system TEP_Final_NoScript/Process Measurements/Subsystem4/Separator Underflow ==
  "       " : Constant  Value=35.3145
  Add : Sum
  Bus Selector : BusSelector  OutputSignals=signal1.FTM(11)
  Bus Selector1 : BusSelector  OutputSignals=XMNS(14)
  XMEAS(14) : Product  Inputs=*//
  "XMEAS(14) " : Outport  VectorParamsAs1DForOutWhenUnconnected=off
  wires:
  "       "/1 -> XMEAS(14)/3
  [DLS] -> XMEAS(14)/2
  [PropertiesStream11] -> Bus Selector/1
  Bus Selector/1 -> XMEAS(14)/1  "<FTM(11)>"
  XMEAS(14)/1 -> Add/1
  Add/1 -> "XMEAS(14) "/1  "XMEAS(14)"
  [XMNS] -> Bus Selector1/1
  Bus Selector1/1 -> Add/2  "<XMNS(14)>"

== system TEP_Final_NoScript/Process Measurements/Subsystem5/Stripper Level ==
  " " : Sum  Inputs=+-
  "    " : Constant  Value=78.25
  "       " : Constant  Value=100
  Add : Sum
  Bus Selector1 : BusSelector  OutputSignals=XMNS(15)
  VTC Total Volume of Stripper ft³ : Constant  Value=156.5
  XMEAS(15) : Product  Inputs=*/*
  "XMEAS(15) " : Outport  VectorParamsAs1DForOutWhenUnconnected=off
  wires:
  " "/1 -> XMEAS(15)/1
  "       "/1 -> XMEAS(15)/3
  "    "/1 -> " "/2
  [VLC] -> " "/1
  VTC Total Volume of Stripper ft³/1 -> XMEAS(15)/2
  XMEAS(15)/1 -> Add/1
  Add/1 -> "XMEAS(15) "/1  "XMEAS(15)"
  [XMNS] -> Bus Selector1/1
  Bus Selector1/1 -> Add/2  "<XMNS(15)>"

== system TEP_Final_NoScript/Process Measurements/Subsystem5/Stripper Pressure ==
  "    " : Constant  Value=760
  "         " : Constant  Value=101.325
  Add : Sum
  Bus Selector1 : BusSelector  OutputSignals=XMNS(16)
  Subtract : Sum  Inputs=+-
  XMEAS(16) : Product  Inputs=*/*
  "XMEAS(16) " : Outport  VectorParamsAs1DForOutWhenUnconnected=off
  wires:
  "    "/1 -> Subtract/2, XMEAS(16)/2
  [PTV] -> Subtract/1
  "         "/1 -> XMEAS(16)/3
  Subtract/1 -> XMEAS(16)/1
  XMEAS(16)/1 -> Add/1
  Add/1 -> "XMEAS(16) "/1  "XMEAS(16)"
  [XMNS] -> Bus Selector1/1
  Bus Selector1/1 -> Add/2  "<XMNS(16)>"

== system TEP_Final_NoScript/Process Measurements/Subsystem5/Stripper Steam Flow ==
  Add : Sum
  Bus Selector1 : BusSelector  OutputSignals=XMNS(19)
  Constant : Constant  Value=0.454
  Constant1 : Constant  Value=1.04E3
  XMEAS(19) : Product  Inputs=3
  "XMEAS(19) " : Outport  VectorParamsAs1DForOutWhenUnconnected=off
  wires:
  Constant1/1 -> XMEAS(19)/2
  [QUC] -> XMEAS(19)/1
  Constant/1 -> XMEAS(19)/3
  XMEAS(19)/1 -> Add/1
  Add/1 -> "XMEAS(19) "/1  "XMEAS(19)"
  [XMNS] -> Bus Selector1/1
  Bus Selector1/1 -> Add/2  "<XMNS(19)>"

== system TEP_Final_NoScript/Process Measurements/Subsystem5/Stripper Temperature ==
  Add : Sum
  Bus Selector1 : BusSelector  OutputSignals=XMNS(18)
  "XMEAS(18) " : Outport  VectorParamsAs1DForOutWhenUnconnected=off
  wires:
  [TCC] -> Add/1
  Add/1 -> "XMEAS(18) "/1  "XMEAS(18)"
  [XMNS] -> Bus Selector1/1
  Bus Selector1/1 -> Add/2  "<XMNS(18)>"

== system TEP_Final_NoScript/Process Measurements/Subsystem5/Stripper Underflow ==
  "       " : Constant  Value=35.3145
  Add : Sum
  Bus Selector : BusSelector  OutputSignals=FTM(13)
  Bus Selector1 : BusSelector  OutputSignals=XMNS(17)
  XMEAS(17) : Product  Inputs=*//
  "XMEAS(17) " : Outport  VectorParamsAs1DForOutWhenUnconnected=off
  wires:
  "       "/1 -> XMEAS(17)/3
  [DLC] -> XMEAS(17)/2
  [PropertiesStream13] -> Bus Selector/1
  Bus Selector/1 -> XMEAS(17)/1  "<FTM(13)>"
  XMEAS(17)/1 -> Add/1
  Add/1 -> "XMEAS(17) "/1  "XMEAS(17)"
  [XMNS] -> Bus Selector1/1
  Bus Selector1/1 -> Add/2  "<XMNS(17)>"

== system TEP_Final_NoScript/Random number generator1/Disturbances I=1-9/Subsystem1 ==
  IDVWLK(2) : Inport
  G : Inport  Port=2
  DIST(2)_0 : Subsystem
  Disturbance calculations I=1-9 : mylib/Disturbance calculations I=1-9  SystemSampleTime=-1  VariantActivationTime=update diagram  AllowFlexibleInterface=on  Latency=0  AutoFrameSizeCalculation=off
      settings: SourceProductName=TEP Library
  Subsystem : Subsystem
      mask Display: color('Blue'),disp('Disturbance constants')
  TESUB8 : mylib/TESUB8  SystemSampleTime=-1  VariantActivationTime=update diagram  AllowFlexibleInterface=on  Latency=0  AutoFrameSizeCalculation=off
      settings: SourceProductName=TEP Library
  TESUB8(2,Time) : Outport  VectorParamsAs1DForOutWhenUnconnected=off
  G_NEW : Outport  Port=2  VectorParamsAs1DForOutWhenUnconnected=off
  wires:
  TESUB8/1 -> TESUB8(2,Time)/1
  Disturbance calculations I=1-9/1 -> TESUB8/1
  Disturbance calculations I=1-9/2 -> G_NEW/1
  IDVWLK(2)/1 -> Disturbance calculations I=1-9/1
  DIST(2)_0/1(DIST) -> Disturbance calculations I=1-9/4
  G/1 -> Disturbance calculations I=1-9/2
  Subsystem/1(Out1) -> Disturbance calculations I=1-9/3

== system TEP_Final_NoScript/Random number generator1/Disturbances I=1-9/Subsystem10 ==
  IDVWLK(1) : Inport
  G : Inport  Port=2
  DIST(1)_0 : Subsystem
  Disturbance calculations I=1-9 : mylib/Disturbance calculations I=1-9  SystemSampleTime=-1  VariantActivationTime=update diagram  AllowFlexibleInterface=on  Latency=0  AutoFrameSizeCalculation=off
      settings: SourceProductName=TEP Library
  Subsystem : Subsystem
      mask Display: color('Blue'),disp('Disturbance constants')
  TESUB8 : mylib/TESUB8  SystemSampleTime=-1  VariantActivationTime=update diagram  AllowFlexibleInterface=on  Latency=0  AutoFrameSizeCalculation=off
      settings: SourceProductName=TEP Library
  TESUB8(1,Time) : Outport  VectorParamsAs1DForOutWhenUnconnected=off
  G_NEW : Outport  Port=2  VectorParamsAs1DForOutWhenUnconnected=off
  wires:
  TESUB8/1 -> TESUB8(1,Time)/1
  Disturbance calculations I=1-9/1 -> TESUB8/1
  Disturbance calculations I=1-9/2 -> G_NEW/1
  IDVWLK(1)/1 -> Disturbance calculations I=1-9/1
  DIST(1)_0/1(DIST) -> Disturbance calculations I=1-9/4
  G/1 -> Disturbance calculations I=1-9/2
  Subsystem/1(Out1) -> Disturbance calculations I=1-9/3

== system TEP_Final_NoScript/Random number generator1/Disturbances I=1-9/Subsystem2 ==
  IDVWLK(3) : Inport
  G : Inport  Port=2
  DIST(3)_0 : Subsystem
  Disturbance calculations I=1-9 : mylib/Disturbance calculations I=1-9  SystemSampleTime=-1  VariantActivationTime=update diagram  AllowFlexibleInterface=on  Latency=0  AutoFrameSizeCalculation=off
      settings: SourceProductName=TEP Library
  Subsystem : Subsystem
      mask Display: color('Blue'),disp('Disturbance constants')
  TESUB8 : mylib/TESUB8  SystemSampleTime=-1  VariantActivationTime=update diagram  AllowFlexibleInterface=on  Latency=0  AutoFrameSizeCalculation=off
      settings: SourceProductName=TEP Library
  TESUB8(3,Time) : Outport  VectorParamsAs1DForOutWhenUnconnected=off
  G_NEW : Outport  Port=2  VectorParamsAs1DForOutWhenUnconnected=off
  wires:
  TESUB8/1 -> TESUB8(3,Time)/1
  Disturbance calculations I=1-9/1 -> TESUB8/1
  Disturbance calculations I=1-9/2 -> G_NEW/1
  IDVWLK(3)/1 -> Disturbance calculations I=1-9/1
  DIST(3)_0/1(DIST) -> Disturbance calculations I=1-9/4
  G/1 -> Disturbance calculations I=1-9/2
  Subsystem/1(Out1) -> Disturbance calculations I=1-9/3

== system TEP_Final_NoScript/Random number generator1/Disturbances I=1-9/Subsystem3 ==
  IDVWLK(4) : Inport
  G : Inport  Port=2
  DIST(4)_0 : Subsystem
  Disturbance calculations I=1-9 : mylib/Disturbance calculations I=1-9  SystemSampleTime=-1  VariantActivationTime=update diagram  AllowFlexibleInterface=on  Latency=0  AutoFrameSizeCalculation=off
      settings: SourceProductName=TEP Library
  Subsystem : Subsystem
      mask Display: color('Blue'),disp('Disturbance constants')
  TESUB8 : mylib/TESUB8  SystemSampleTime=-1  VariantActivationTime=update diagram  AllowFlexibleInterface=on  Latency=0  AutoFrameSizeCalculation=off
      settings: SourceProductName=TEP Library
  TESUB8(4,Time) : Outport  VectorParamsAs1DForOutWhenUnconnected=off
  G_NEW : Outport  Port=2  VectorParamsAs1DForOutWhenUnconnected=off
  wires:
  TESUB8/1 -> TESUB8(4,Time)/1
  Disturbance calculations I=1-9/1 -> TESUB8/1
  Disturbance calculations I=1-9/2 -> G_NEW/1
  IDVWLK(4)/1 -> Disturbance calculations I=1-9/1
  DIST(4)_0/1(DIST) -> Disturbance calculations I=1-9/4
  G/1 -> Disturbance calculations I=1-9/2
  Subsystem/1(Out1) -> Disturbance calculations I=1-9/3

== system TEP_Final_NoScript/Random number generator1/Disturbances I=1-9/Subsystem4 ==
  IDVWLK(5) : Inport
  G : Inport  Port=2
  DIST(5)_0 : Subsystem
  Disturbance calculations I=1-9 : mylib/Disturbance calculations I=1-9  SystemSampleTime=-1  VariantActivationTime=update diagram  AllowFlexibleInterface=on  Latency=0  AutoFrameSizeCalculation=off
      settings: SourceProductName=TEP Library
  Subsystem : Subsystem
      mask Display: color('Blue'),disp('Disturbance constants')
  TESUB8 : mylib/TESUB8  SystemSampleTime=-1  VariantActivationTime=update diagram  AllowFlexibleInterface=on  Latency=0  AutoFrameSizeCalculation=off
      settings: SourceProductName=TEP Library
  TESUB8(5,Time) : Outport  VectorParamsAs1DForOutWhenUnconnected=off
  G_NEW : Outport  Port=2  VectorParamsAs1DForOutWhenUnconnected=off
  wires:
  TESUB8/1 -> TESUB8(5,Time)/1
  Disturbance calculations I=1-9/1 -> TESUB8/1
  Disturbance calculations I=1-9/2 -> G_NEW/1
  IDVWLK(5)/1 -> Disturbance calculations I=1-9/1
  DIST(5)_0/1(DIST) -> Disturbance calculations I=1-9/4
  Subsystem/1(Out1) -> Disturbance calculations I=1-9/3
  G/1 -> Disturbance calculations I=1-9/2

== system TEP_Final_NoScript/Random number generator1/Disturbances I=1-9/Subsystem5 ==
  IDVWLK(6) : Inport
  G : Inport  Port=2
  DIST(6)_0 : Subsystem
  Disturbance calculations I=1-9 : mylib/Disturbance calculations I=1-9  SystemSampleTime=-1  VariantActivationTime=update diagram  AllowFlexibleInterface=on  Latency=0  AutoFrameSizeCalculation=off
      settings: SourceProductName=TEP Library
  Subsystem : Subsystem
      mask Display: color('Blue'),disp('Disturbance constants')
  TESUB8 : mylib/TESUB8  SystemSampleTime=-1  VariantActivationTime=update diagram  AllowFlexibleInterface=on  Latency=0  AutoFrameSizeCalculation=off
      settings: SourceProductName=TEP Library
  TESUB8(6,Time) : Outport  VectorParamsAs1DForOutWhenUnconnected=off
  G_NEW : Outport  Port=2  VectorParamsAs1DForOutWhenUnconnected=off
  wires:
  TESUB8/1 -> TESUB8(6,Time)/1
  Disturbance calculations I=1-9/1 -> TESUB8/1
  Disturbance calculations I=1-9/2 -> G_NEW/1
  IDVWLK(6)/1 -> Disturbance calculations I=1-9/1
  DIST(6)_0/1(DIST) -> Disturbance calculations I=1-9/4
  G/1 -> Disturbance calculations I=1-9/2
  Subsystem/1(Out1) -> Disturbance calculations I=1-9/3

== system TEP_Final_NoScript/Random number generator1/Disturbances I=1-9/Subsystem6 ==
  IDVWLK(7) : Inport
  G : Inport  Port=2
  DIST(7)_0 : Subsystem
  Disturbance calculations I=1-9 : mylib/Disturbance calculations I=1-9  SystemSampleTime=-1  VariantActivationTime=update diagram  AllowFlexibleInterface=on  Latency=0  AutoFrameSizeCalculation=off
      settings: SourceProductName=TEP Library
  Subsystem : Subsystem
      mask Display: color('Blue'),disp('Disturbance constants')
  TESUB8 : mylib/TESUB8  SystemSampleTime=-1  VariantActivationTime=update diagram  AllowFlexibleInterface=on  Latency=0  AutoFrameSizeCalculation=off
      settings: SourceProductName=TEP Library
  TESUB8(7,Time) : Outport  VectorParamsAs1DForOutWhenUnconnected=off
  G_NEW : Outport  Port=2  VectorParamsAs1DForOutWhenUnconnected=off
  wires:
  TESUB8/1 -> TESUB8(7,Time)/1
  Disturbance calculations I=1-9/1 -> TESUB8/1
  IDVWLK(7)/1 -> Disturbance calculations I=1-9/1
  G/1 -> Disturbance calculations I=1-9/2
  Subsystem/1(Out1) -> Disturbance calculations I=1-9/3
  DIST(7)_0/1(DIST) -> Disturbance calculations I=1-9/4
  Disturbance calculations I=1-9/2 -> G_NEW/1

== system TEP_Final_NoScript/Random number generator1/Disturbances I=1-9/Subsystem7 ==
  IDVWLK(8) : Inport
  G : Inport  Port=2
  DIST(8)_0 : Subsystem
  Disturbance calculations I=1-9 : mylib/Disturbance calculations I=1-9  SystemSampleTime=-1  VariantActivationTime=update diagram  AllowFlexibleInterface=on  Latency=0  AutoFrameSizeCalculation=off
      settings: SourceProductName=TEP Library
  Subsystem : Subsystem
      mask Display: color('Blue'),disp('Disturbance constants')
  TESUB8 : mylib/TESUB8  SystemSampleTime=-1  VariantActivationTime=update diagram  AllowFlexibleInterface=on  Latency=0  AutoFrameSizeCalculation=off
      settings: SourceProductName=TEP Library
  TESUB8(8,Time) : Outport  VectorParamsAs1DForOutWhenUnconnected=off
  G_NEW : Outport  Port=2  VectorParamsAs1DForOutWhenUnconnected=off
  wires:
  TESUB8/1 -> TESUB8(8,Time)/1
  Disturbance calculations I=1-9/1 -> TESUB8/1
  Disturbance calculations I=1-9/2 -> G_NEW/1
  IDVWLK(8)/1 -> Disturbance calculations I=1-9/1
  G/1 -> Disturbance calculations I=1-9/2
  Subsystem/1(Out1) -> Disturbance calculations I=1-9/3
  DIST(8)_0/1(DIST) -> Disturbance calculations I=1-9/4

== system TEP_Final_NoScript/Random number generator1/Disturbances I=1-9/Subsystem8 ==
  IDVWLK(9) : Inport
  G : Inport  Port=2
  DIST(9)_0 : Subsystem
  Disturbance calculations I=1-9 : mylib/Disturbance calculations I=1-9  SystemSampleTime=-1  VariantActivationTime=update diagram  AllowFlexibleInterface=on  Latency=0  AutoFrameSizeCalculation=off
      settings: SourceProductName=TEP Library
  Subsystem : Subsystem
      mask Display: color('Blue'),disp('Disturbance constants')
  TESUB8 : mylib/TESUB8  SystemSampleTime=-1  VariantActivationTime=update diagram  AllowFlexibleInterface=on  Latency=0  AutoFrameSizeCalculation=off
      settings: SourceProductName=TEP Library
  TESUB8(9,Time) : Outport  VectorParamsAs1DForOutWhenUnconnected=off
  G_NEW : Outport  Port=2  VectorParamsAs1DForOutWhenUnconnected=off
  wires:
  TESUB8/1 -> TESUB8(9,Time)/1
  Disturbance calculations I=1-9/1 -> TESUB8/1
  Disturbance calculations I=1-9/2 -> G_NEW/1
  IDVWLK(9)/1 -> Disturbance calculations I=1-9/1
  G/1 -> Disturbance calculations I=1-9/2
  Subsystem/1(Out1) -> Disturbance calculations I=1-9/3
  DIST(9)_0/1(DIST) -> Disturbance calculations I=1-9/4
